simulink model "GreenCraneModel_Adjusted_110225"  (R2024b)
settings: Solver=VariableStepAuto  StartTime=0.0  StopTime=60  RelTol=1e-5
model workspace (MATLAB code in the model file):
  | %% hydralic
  | %liqud data
  | rho_l = 850;
  | 
  | %Pressure
  | Ps = 108; %bar
  | 
  | %valve data
  | pRat = 30e5; %rated pressure
  | Cd = 0.6; %discarge coefficient
  | QRat = 270/6e4;
  | Admax = QRat/Cd/(2/rho_l*pRat/2)^0.5;
  | %% multibody
  | %Cylinder 1
  | sC_1 = 0.45; %Stroke
  | L0C_1 = 0.4; %Deadlength
  | x0C_1 = 0.0; %Initial position
  | dC_1 = 0.065; %Piston diameter
  | dRC_1 = 0.035; %Rod diameter
  | %Derived values
  | dOC_1 = dC_1 + dC_1/4; %Cylinder outer diameter
  | LC_1 = sC_1 + L0C_1/3; %Cylinder length
  | tEPC_1 = L0C_1/6; %Thickness of end plate
  | dJC_1 = L0C_1/3; %Diameter of joint
  | LJC_1 = dRC_1; %Length of joint
  | LRC_1 = sC_1 + tEPC_1; %Length of rod
  | tPC_1 = L0C_1/3; %Thickness of piston
  | AC_1 = pi*dC_1^2/4; %Piston area
  | ARC_1 = pi*dRC_1^2/4; %Rod area
  | AAC_1 = AC_1 - ARC_1; %Annulus area
  | Initial_Pos = x0C_1-0.116;
  | 
  | % crane arm
  | g=9.81;
  | theta1_init=0*pi/180;
  | thetaDot1_init=0;
  | L1=3.625;
  | rho=7800;
  | L4 = 0.229;
  | Lg4x = L1-L4/2;
  | Lg4y = 0.08157;
  | 
  | abx = 0.730-0.100-0.080; %0.550; %730-100-80
  | aby = (0.223-0.075); %-0.130; %0.223-75
  | g = 9.81;
  | G1 =100*g;
  | G4 = (4*76+16)*g;
  | 
  | G = 440*g; %440*g; %447.10945
  | Gx = 3.03499; %3.03499; %3.03499
  | Gy = 0.140; %0.2; %0.06071
  | 
  | Cy = -1.040;
  | Cx = 0.427;
  | ang_CA = atan2(Cy,Cx);
  | ang_k = atan2(aby,abx);
  | b = abs(sqrt(Cy^2+Cx^2));
  | c = abs(sqrt(abx^2+aby^2)); %56.73
  | % FBD Calculations
  | %syms Ax Ay P gamma beta ang_C ang_AB r_cb r_ab L3(i) w_A w_C VBx VBy Vp crs_abp
  | L3_min = 0.772;
  | L3 = L3_min+Initial_Pos; %0.5*(x-1)/(1000-1) + 0.772;  %.172*sin(X)/1 + 0.772+0.175 0;
  | 
  | ang_C = acos((L3^2+b^2-c^2)/(2*L3*b));
  | beta = ang_CA + pi - ang_C;
  | 
  | bx = L3*cos(beta) + Cx;
  | by = L3*sin(beta) + Cy;
  | ang_AB =atan2(by,bx);
  | gamma = ang_AB + ang_k;
  | 
  | r_cb = [L3*cos(beta);L3*sin(beta);0];
  | r_ab = [bx; by; 0 ];
  | 
  | 
  | crs_abp = cross(r_ab, [cos(beta); sin(beta);0]);
  | matrix = [1, 0, cos(beta);
  |           0, 1, sin(beta);
  |           0, 0, r_ab(1)*sin(beta) - r_ab(2)*cos(beta)];
  | right = [0;(G1+G4);G*(Gx*cos(gamma)-Gy*sin(gamma))];%(G1*cos(gamma)*L1/2+G4*(cos(gamma)*Lg4x-sin(gamma)*Lg4y))
  | 
  | ANS = inv(matrix)*right;
  | Ax = ANS(1);
  | Ay = ANS(2);
  | Fl  = ANS(3); %N
  | 
  | 
  | %% FF
  | dP_0 = 7e5; %Pressure drop with comp
  | phi = 0.7130;
  | A = AC_1; % Area piston side
  | Ar = AAC_1; % Area rod side
  | BW = 0; % deadband
  | SpoolTravel = 7; % Maximum Spool Travel
  | a = (SpoolTravel-BW)/25; % Valve Slope Characteristic [mm/(L/min)]
  | 
  | %deadband
  | DeadUp = 0.13;
  | DeadDown = 0.12;
  | 
  | %% Friction force from script
  |    F_friction = 1133.4; %N
  | 
  | %% Spool travel
  | 
  | 
  | 
  | % Down
  |     U_down_vec = [0, DeadDown ,0.2, 0.4, 0.6, 0.7, 0.8, 1.0];
  |     K_down = [1e-5,1e-5,0.75,2.17,3.39,3.99,4.55,4.84]/(6e4 * sqrt(1e5));
  |     Ad_down = (K_down/(Cd*sqrt(2/rho_l))) *1e6; %mm^2
  |     Ad_down2 = 1.5*Ad_down;
  |     Ad_max_PA = 8.76; %mm^2
  |     Ad_max_BT = 1.2*Ad_max_PA;
  |     Ad_max_PB = 8.76; %mm^2
  |     Ad_max_AT = Ad_max_PB;
  | %     Dp_down_vec = [21.20, 32.96, 43.85, 48.10, 60.36]*1e5; %Pa pressure drop
  | %     VFR_down = [-3.55, -4.47, -5.18, -5.62, -6.191;
  | %            -9.95, -12.14, -14.83, -15.42, -18.60;
  | %            -14.10, -18.67, -22.17, -23.27, -27.33;
  | %            -16.96, -22.28, -27.57, -27.55, -33.1;
  | %            -17.88, -23.71, -29.04, -31.04, -35.92;
  | %            -20.53, -26.74, -32.73, -35.00, -37.53]/6e4; %m^3/s Flow
  | %     for i = 1:length(Dp_down_vec)
  | %         for j = 1:length(U_down_vec)
  | %         OAV_6x5 = sqrt( (VFR_down(i,j)).^2./(Cd^2*Dp_down_vec(i)*2/rho_l)  );
  | %         end
  | %     end
  | %
  | %
  | % % Up
  |     U_up_vec = [0, DeadUp ,0.2, 0.4, 0.6, 0.7, 0.8, 1.0];
  |     K_up = [1e-5,1e-5,0.78,2.29,3.42,4.59,5.09,5.71]/(6e4 * sqrt(1e5));
  |     Ad_up = (K_up/(Cd*sqrt(2/rho_l))) *1e6; %mm^2
  | %     Dp_up_vec = [17.39, 28.25, 36.01, 42.60, 56.50];
  | %     VFR_up = [3.36, 4.38, 4.90, 5.43, 5.86;
  | %               10.08, 12.24, 14.15, 15.51, 18.16;
  | %               9.25, 18.98, 22.92, 24.74, 27.65;
  | %               19.56, 24.95, 26.61, 29.47, 34.19;
  | %               14.84, 26.72, 32.17, 33.89, 38.51;
  | %               24.92, 26.56, 34.56, 38.50, 37.29];
  | %
  | 
  | %% motion ref
  | Amp = 0.1;
  | Mean = Amp;
values from neighbouring files (symbols this model uses):
  N = [Fl-Ffr ... (first row only)    [fyske_parametere.m]
  X = X_data.("<fPistonPosition_G_OPCfPistonPosition>")    [friksjon.m]    (also in fyske_parametere.m = M\N)
undefined symbols (not defined in the file or in its folder): Y, Z
libraries: sm_lib x35, fl_lib x31, nesl_utility x23, SimscapeFluids_lib x10, slpidlib x1
(part 1 of 3)
settings Model: Creator=Emila  LastModifiedBy=Emil
settings RTWCC: GPUComputeCapability=3.5
settings ConfigComp: PLC_OutputDir=Skrivebord  PLC_TargetIDE=twincat3  PLC_MultiTBSigbuilderTimeRange=off  PLC_FoldFBCallOutputVar=off  PLC_RemoveUnusedSSMethodCallArguments=off  PLC_UseCallOutputArgSyntax=off  PLC_EnableUnsignedAndDoubleTypes=off  PLC_EnableUDTSplitting=off  PLC_MaxFieldsInUDT=500  PLC_InlineEnumCastFunction=off

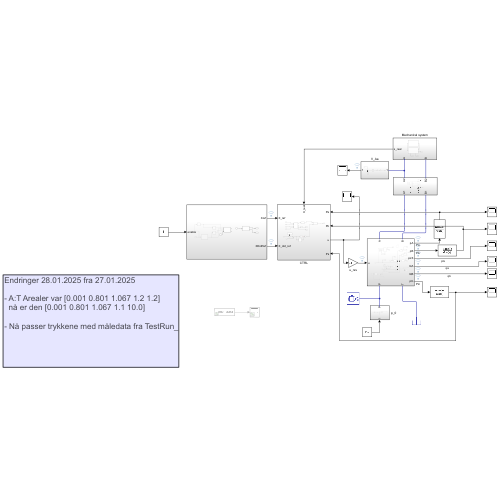
[thumbnail: Simulink's stored preview of the top-level diagram]
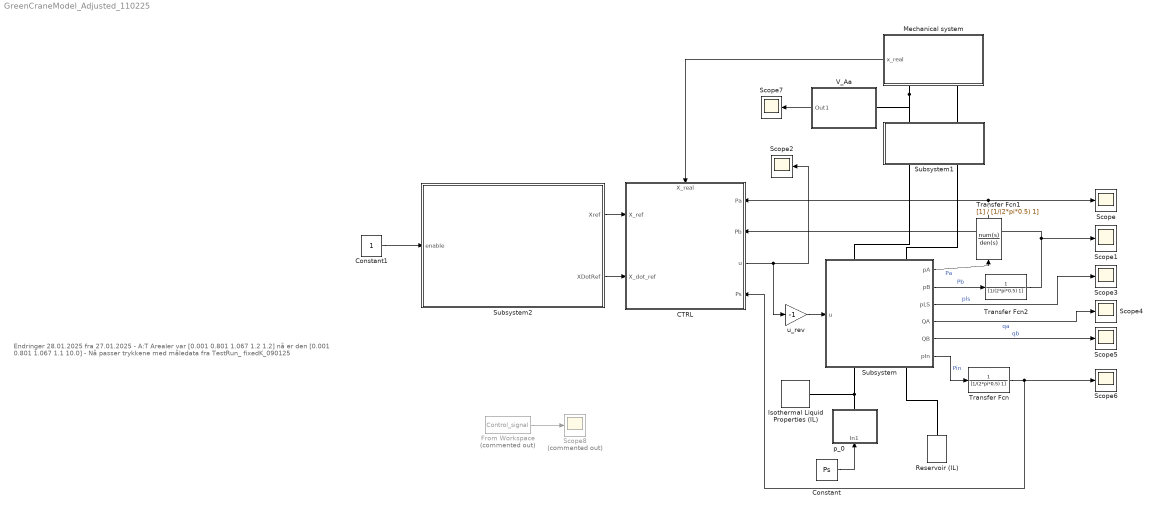
== system GreenCraneModel_Adjusted_110225 ==
  note: Endringer 28.01.2025 fra 27.01.2025
      |
      | - A:T Arealer var [0.001 0.801 1.067 1.2 1.2]
      |   nå er den [0.001 0.801 1.067 1.1 10.0]
      |
      | - Nå passer trykkene med måledata fra TestRun_ fixedK_090125
  CTRL : Subsystem
      settings: PortSchema="{\"entries\":[{\"content\":{\"sides\":[{\"content\":{\"connectorIds\":[\"In1\",\"In2\"]},\"type\":\"ConnectorPlacement.EquallySpacedRectSide\",\"uuid\":\"e7dc98bc-0c39-42fc-9d44-5c528a861935\"},{\"content\":{\"connectorIds\":[\"In4\",\"In5\",\"Out1\",\"In6\"],\"side\":\"RIGHT\"},\"type\":\"ConnectorPlacement.EquallySpacedRectSide\",\"uuid\":\"7a7fb2e4-7f4e-4840-80a8-3a9723ecfbf6\"},{\"content\":{\"connectorIds\":[\"In3\"],\"side\":\"TOP\"},\"type\":\"ConnectorPlacement.EquallySpacedRectSide\",\"uuid\":\"8314552e-40ce-493a-a910-ea6a3ee6c4fc\"}]},\"type\":\"ConnectorPlacement.EquallySpacedConnector\",\"uuid\":\"904788e7-187d-4514-a00a-56ca1dbc298c\"}],\"packageUris\":[\"http://schema.mathworks.com/mf0/Connector/R2020b\"],\"version\":\"1.0\"}"
  Constant : Constant  Value=Ps
  Constant1 : Constant
  From Workspace : FromWorkspace  Commented=on  VariableName=Control_signal  SampleTime=-1
  Isothermal Liquid Properties (IL) : fl_lib/Isothermal Liquid/Utilities/Isothermal Liquid Properties (IL)  rho_L_atm=rho_l kg/m^3  bulk_modulus_model=foundation.enum.bulk_modulus_model.const  beta_gain=6  beta_L_atm=2.1791e9 Pa  nu_atm=1.0034e-6 m^2/s  p_atm=0.101325 MPa  p_min=1 Pa  properties_range_check=simscape.enum.assert.action.error  air_fraction=0.005  polytropic_index=1.0  rho_g_atm=1.225 kg/m^3  air_dissolution_model=false  p_crit=3 MPa
  Mechanical system : Subsystem
      settings: PortSchema="{\"entries\":[{\"content\":{\"sides\":[{\"content\":{},\"type\":\"ConnectorPlacement.EquallySpacedRectSide\",\"uuid\":\"e7d79fdb-c1af-44b7-bd08-96b300e6958a\"},{\"content\":{\"connectorIds\":[\"RConn1\",\"RConn2\"],\"side\":\"RIGHT\"},\"type\":\"ConnectorPlacement.EquallySpacedRectSide\",\"uuid\":\"9182fec9-179c-4b8b-a801-95a4bf7282c9\"},{\"content\":{\"connectorIds\":[\"Out1\"],\"side\":\"TOP\"},\"type\":\"ConnectorPlacement.EquallySpacedRectSide\",\"uuid\":\"910325c5-b244-4f4d-b947-94cfd0509a86\"}]},\"type\":\"ConnectorPlacement.EquallySpacedConnector\",\"uuid\":\"3b4ea8e7-81a3-45c9-bfcb-55ef2a8eba89\"}],\"packageUris\":[\"http://schema.mathworks.com/mf0/Connector/R2020b\"],\"version\":\"1.0\"}"
  Reservoir (IL) : fl_lib/Isothermal Liquid/Elements/Reservoir (IL)  reservoir_type=foundation.enum.constant_controlled.constant  pressure_spec=foundation.enum.pressure_spec.atmospheric  reservoir_pressure=0.101325 MPa
  Scope{,1..7} (8 alike) : Scope
  Scope8 : Scope  Commented=on
  Subsystem : Subsystem
      settings: PortSchema="{\"entries\":[{\"content\":{\"sides\":[{\"content\":{\"connectorIds\":[\"In1\"]},\"type\":\"ConnectorPlacement.EquallySpacedRectSide\",\"uuid\":\"2106b7c6-6d92-4a39-9b3d-8951ce8b04e8\"},{\"content\":{\"connectorIds\":[\"Out1\",\"Out2\",\"Out3\",\"Out4\",\"Out5\",\"Out6\"],\"side\":\"RIGHT\"},\"type\":\"ConnectorPlacement.EquallySpacedRectSide\",\"uuid\":\"760f4e6f-1347-4e69-a63e-1f73879098bb\"},{\"content\":{\"connectorIds\":[\"LConn1\",\"LConn2\"],\"side\":\"TOP\"},\"type\":\"ConnectorPlacement.EquallySpacedRectSide\",\"uuid\":\"9e6a4ebb-fb50-453b-b1c2-4c0835e6495a\"},{\"content\":{\"connectorIds\":[\"RConn1\",\"RConn2\"],\"side\":\"BOTTOM\"},\"type\":\"ConnectorPlacement.EquallySpacedRectSide\",\"uuid\":\"fda93e11-89cc-40b0-95ae-4a4fae923076\"}]},\"type\":\"ConnectorPlacement.EquallySpacedConnector\",\"uuid\":\"37d72eb9-77aa-495f-a16f-a1eebb071270\"}],\"packageUris\":[\"http://schema.mathworks.com/mf0/Connector/R2020b\"],\"version\":\"1.0\"}"
  Subsystem1 : Subsystem
      settings: PortSchema="{\"entries\":[{\"content\":{\"sides\":[{\"content\":{},\"type\":\"ConnectorPlacement.EquallySpacedRectSide\",\"uuid\":\"a9f0eaf7-f148-41af-883d-8aedf66e3fe7\"},{\"content\":{\"side\":\"RIGHT\"},\"type\":\"ConnectorPlacement.EquallySpacedRectSide\",\"uuid\":\"b7d06a0e-217c-4594-9653-b1704beb7fcf\"},{\"content\":{\"connectorIds\":[\"LConn1\",\"LConn2\"],\"side\":\"TOP\"},\"type\":\"ConnectorPlacement.EquallySpacedRectSide\",\"uuid\":\"8b0b6e4d-8977-4f79-be82-c14ccdce2671\"},{\"content\":{\"connectorIds\":[\"RConn1\",\"RConn2\"],\"side\":\"BOTTOM\"},\"type\":\"ConnectorPlacement.EquallySpacedRectSide\",\"uuid\":\"d5bd5d30-b17c-4999-a2e1-ca2e0a57ee34\"}]},\"type\":\"ConnectorPlacement.EquallySpacedConnector\",\"uuid\":\"f712f636-cf3b-4e26-b860-5f0ebbe71685\"}],\"packageUris\":[\"http://schema.mathworks.com/mf0/Connector/R2020b\"],\"version\":\"1.0\"}"
  Subsystem2 : Subsystem
  Transfer Fcn : TransferFcn  Denominator=[1/(2*pi*0.5) 1]
  Transfer Fcn1 : TransferFcn  Denominator=[1/(2*pi*0.5) 1]
  Transfer Fcn2 : TransferFcn  Denominator=[1/(2*pi*0.5) 1]
  V_Aa : Subsystem
  p_0 : Subsystem
      settings: PortSchema="{\"entries\":[{\"content\":{\"sides\":[{\"content\":{\"connectorIds\":[\"LConn1\"]},\"type\":\"ConnectorPlacement.EquallySpacedRectSide\",\"uuid\":\"c4662dc8-9dce-4e03-a503-caebb8aa604d\"},{\"content\":{\"connectorIds\":[\"In1\"],\"side\":\"RIGHT\"},\"type\":\"ConnectorPlacement.EquallySpacedRectSide\",\"uuid\":\"29be6a65-4201-4b09-abee-03d6b9c83b9e\"},{\"content\":{\"side\":\"TOP\"},\"type\":\"ConnectorPlacement.EquallySpacedRectSide\",\"uuid\":\"b7c22780-7148-4981-a76e-0df66b5436d6\"},{\"content\":{\"side\":\"BOTTOM\"},\"type\":\"ConnectorPlacement.EquallySpacedRectSide\",\"uuid\":\"0d33656d-2c34-499b-a6f6-06036ba0bd38\"}]},\"type\":\"ConnectorPlacement.EquallySpacedConnector\",\"uuid\":\"6213fc7c-057e-48b9-b0cb-4c92532ae427\"}],\"packageUris\":[\"http://schema.mathworks.com/mf0/Connector/R2020b\"],\"version\":\"1.0\"}"
  u_rev : Gain  Gain=-1
  wires:
  V_Aa/1(Out1) -> Scope7/1
  Subsystem/1(pA) -> Transfer Fcn1/1  "Pa"
  Constant/1 -> p_0/1(In1)
  Subsystem/2(pB) -> Transfer Fcn2/1  "Pb"
  CTRL/1(u) -> Scope2/1, u_rev/1
  Subsystem/6(pIn) -> Transfer Fcn/1  "Pin"
  Mechanical system/1(x_real) -> CTRL/3(X_real)
  Subsystem/3(pLS) -> Scope3/1  "pls"
  Subsystem/5(QB) -> Scope5/1  "qb"
  Subsystem/4(QA) -> Scope4/1  "qa"
  Transfer Fcn/1 -> CTRL/6(Ps), Scope6/1
  Transfer Fcn2/1 -> CTRL/5(Pb), Scope1/1
  Transfer Fcn1/1 -> CTRL/4(Pa), Scope/1
  Subsystem2/1(Xref) -> CTRL/1(X_ref)
  Subsystem2/2(XDotRef) -> CTRL/2(X_dot_ref)
  Constant1/1 -> Subsystem2/1(enable)
  u_rev/1 -> Subsystem/1(u)
  From Workspace/1 -> Scope8/1
  connections:
  Mechanical system/RConn1 -- Subsystem1/LConn1 -- V_Aa/LConn1
  p_0/LConn1 -- Subsystem/RConn1 -- Isothermal Liquid Properties (IL)/RConn1
  Subsystem/LConn1 -- Subsystem1/RConn1
  Subsystem/LConn2 -- Subsystem1/RConn2
  Subsystem1/LConn2 -- Mechanical system/RConn2
  Reservoir (IL)/LConn1 -- Subsystem/RConn2

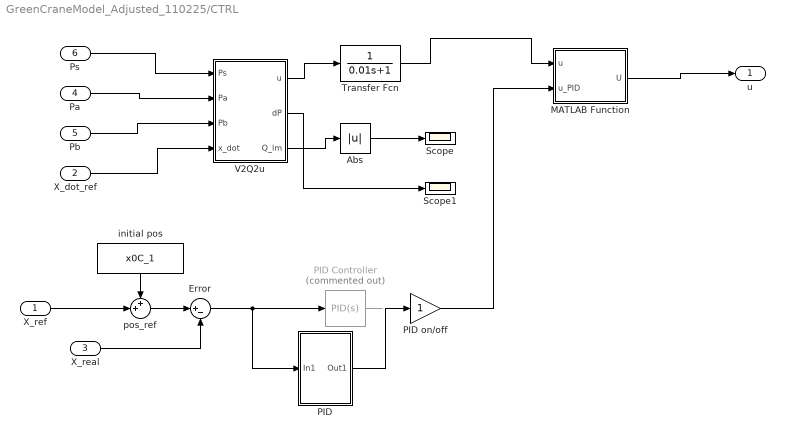
== system GreenCraneModel_Adjusted_110225/CTRL ==
  X_ref : Inport
  X_dot_ref : Inport  Port=2
  X_real : Inport  Port=3
  Pa : Inport  Port=4
  Pb : Inport  Port=5
  Ps : Inport  Port=6
  Abs : Abs  SaturateOnIntegerOverflow=off
  Error : Sum  Inputs=|+-
  MATLAB Function : MATLAB Function  TreatAsAtomicUnit=on
  PID : Subsystem
  PID Controller : slpidlib/PID Controller  Commented=on  Controller=PID  Form=Parallel  TimeDomain=Continuous-time  UseExternalTs=off  SampleTime=-1  IntegratorMethod=Forward Euler  FilterMethod=Forward Euler  ControllerParametersSource=internal  P=5  I=1  UseKiTs=off  D=1  UseExternalDerivativeSource=off  N=1e10  UseFilter=on  TunerSelectOption=Transfer Function Based (PID Tuner App)  InitialConditionSource=internal  InitialConditionForIntegrator=0  InitialConditionForFilter=0  DifferentiatorICPrevScaledInput=0  ExternalReset=none  TrackingMode=off  Kt=1  LimitOutput=off  SatLimitsSource=internal  UpperSaturationLimit=inf  LowerSaturationLimit=-inf  LinearizeAsGain=on  AntiWindupMode=none  Kb=1  LimitIntegrator=off  UpperIntegratorSaturationLimit=inf  LowerIntegratorSaturationLimit=-inf  POutMin=[]  POutMax=[]  IOutMin=[]  IOutMax=[]  DOutMin=[]  DOutMax=[]  NOutMin=[]  NOutMax=[]  SumOutMin=[]  SumOutMax=[]  SaturationOutMin=[]  SaturationOutMax=[]  PParamMin=[]  PParamMax=[]  IParamMin=[]  IParamMax=[]  DParamMin=[]  DParamMax=[]  NParamMin=[]  NParamMax=[]  KbParamMin=[]  KbParamMax=[]  KtParamMin=[]  KtParamMax=[]  KbOutMin=[]  KbOutMax=[]  KtOutMin=[]  KtOutMax=[]  IntegratorOutMin=[]  IntegratorOutMax=[]  FilterOutMin=[]  FilterOutMax=[]  SumI1OutMin=[]  SumI1OutMax=[]  SumI2OutMin=[]  SumI2OutMax=[]  SumI3OutMin=[]  SumI3OutMax=[]  SumI4OutMin=[]  SumI4OutMax=[]  SumDOutMin=[]  SumDOutMax=[]  DifferentiatorOutMin=[]  DifferentiatorOutMax=[]  FilterDiffOutCoefMin=[]  FilterDiffOutCoefMax=[]  ReciprocalOutMin=[]  ReciprocalOutMax=[]  SumDenOutMin=[]  SumDenOutMax=[]  SumNumOutMin=[]  SumNumOutMax=[]  DivideOutMin=[]  DivideOutMax=[]  UdiffTsProdOutMin=[]  UdiffTsProdOutMax=[]  NTsProdOutMin=[]  NTsProdOutMax=[]  UintegralTsProdOutMin=[]  UintegralTsProdOutMax=[]  UngainTsProdOutMin=[]  UngainTsProdOutMax=[]  ClampingZeroOutDataTypeStr=Inherit: Inherit via back propagation  ClampingZeroOutMin=[]  ClampingZeroOutMax=[]  FilterDenConstantOutDataTypeStr=Inherit: Inherit via back propagation  FilterDenConstantOutMin=[]  FilterDenConstantOutMax=[]  PCopyOutDataTypeStr=Inherit: Inherit via back propagation  PCopyOutMin=[]  PCopyOutMax=[]  NCopyOutDataTypeStr=Inherit: Inherit via back propagation  NCopyOutMin=[]  NCopyOutMax=[]  IntegratorContinuousStateAttributes=''  IntegratorStateMustResolveToSignalObject=off  IntegratorRTWStateStorageClass=Auto  FilterContinuousStateAttributes=''  FilterStateMustResolveToSignalObject=off  FilterRTWStateStorageClass=Auto  ParallelPVariant=InternalParameters  IdealPVariant=Disabled  IVariant=InternalParameters  DVariant=InternalParameters  IntegratorVariant=Continuous  SatVariant=Disabled  AWVariant=Passthrough  PCopyVariant=Disabled  TRVariant=Disabled  FdbkBlocksVariant=Forward  IdealPFdbkVariant=Disabled  SatFdbkVariant=Disabled  DerivativeFilterVariant=ContFilter  NVariant=InternalParameters  NCopyVariant=Disabled  FilterICVariant=InternalICsFilter  IntegratorICVariant=InternalICs  ExternalResetVariant=Disabled  TRSumVariant=Passthrough  SumFdbkVariant=Disabled  SumVariant=Sum_PID  TsampFilterVariant=InternalTs  TsampNgainVariant=Passthrough  TsampIntegralVariant=Disabled_SignalSpec  ExternalSaturationOutDataTypeStr=Inherit: Same as second input  DerivativeSourceVariant=ErrorSignal  PreIntVariant=InternalPreInt
  PID on/off : Gain
  Scope : Scope
  Scope1 : Scope
  Transfer Fcn : TransferFcn  Denominator=[0.01 1]
  V2Q2u : MATLAB Function  TreatAsAtomicUnit=on
  initial pos : Constant  Value=x0C_1
  pos_ref : Sum  Inputs=++|
  u : Outport
  wires:
  X_real/1 -> Error/2
  Pb/1 -> V2Q2u/3(Pb)
  Pa/1 -> V2Q2u/2(Pa)
  Ps/1 -> V2Q2u/1(Ps)
  V2Q2u/3(Q_lm) -> Abs/1
  V2Q2u/2(dP) -> Scope1/1
  X_ref/1 -> pos_ref/2
  pos_ref/1 -> Error/1
  initial pos/1 -> pos_ref/1
  V2Q2u/1(u) -> Transfer Fcn/1
  Abs/1 -> Scope/1
  PID Controller/1 -> ?
  Transfer Fcn/1 -> MATLAB Function/1(u)
  MATLAB Function/1(U) -> u/1
  PID/1(Out1) -> PID on/off/1
  Error/1 -> PID/1(In1), PID Controller/1
  X_dot_ref/1 -> V2Q2u/4(x_dot)
  PID on/off/1 -> MATLAB Function/2(u_PID)

== system GreenCraneModel_Adjusted_110225/Mechanical system ==
  Cylinder_1 : Subsystem
      settings: PortSchema="{\"entries\":[{\"content\":{\"sides\":[{\"content\":{\"connectorIds\":[\"LConn1\"]},\"type\":\"ConnectorPlacement.EquallySpacedRectSide\",\"uuid\":\"0d78c50f-9421-405f-914f-ba400f0edc4e\"},{\"content\":{\"connectorIds\":[\"RConn1\",\"Out1\"],\"side\":\"RIGHT\"},\"type\":\"ConnectorPlacement.EquallySpacedRectSide\",\"uuid\":\"3613fe88-8080-4676-8b90-d4f5ec3e9571\"},{\"content\":{\"side\":\"TOP\"},\"type\":\"ConnectorPlacement.EquallySpacedRectSide\",\"uuid\":\"fa977bd5-6674-458e-9bf8-be2185a48584\"},{\"content\":{\"connectorIds\":[\"RConn2\",\"RConn3\"],\"side\":\"BOTTOM\"},\"type\":\"ConnectorPlacement.EquallySpacedRectSide\",\"uuid\":\"b9e74392-c07a-48b0-8e27-d5ae7d883bf0\"}]},\"type\":\"ConnectorPlacement.EquallySpacedConnector\",\"uuid\":\"3e102c0d-02bf-4808-a7bf-f6d405498545\"}],\"packageUris\":[\"http://schema.mathworks.com/mf0/Connector/R2020b\"],\"version\":\"1.0\"}"
  mechanical system : Subsystem
  A : PMIOPort  Side=Right
  B : PMIOPort  Port=2  Side=Right
  x_real : Outport
  wires:
  Cylinder_1/1(x_real) -> x_real/1
  connections:
  mechanical system/LConn1 -- Cylinder_1/LConn1
  mechanical system/RConn1 -- Cylinder_1/RConn1
  B/RConn1 -- Cylinder_1/RConn3
  A/RConn1 -- Cylinder_1/RConn2

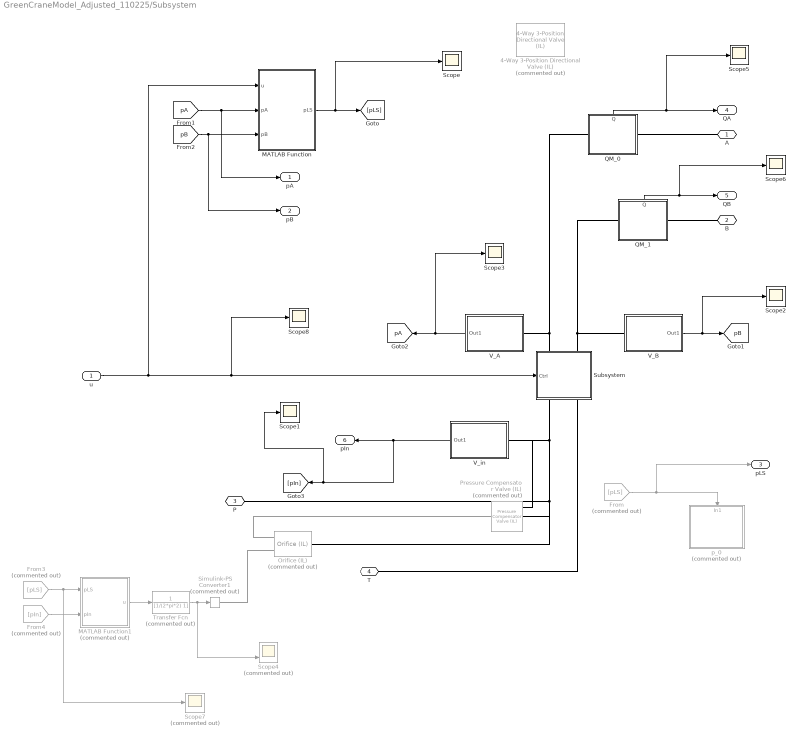
== system GreenCraneModel_Adjusted_110225/Subsystem ==
  u : Inport
  4-Way 3-Position Directional Valve (IL) : SimscapeFluids_lib/Isothermal Liquid/Valves & Orifices/Directional Control Valves/4-Way 3-Position Directional Valve (IL)  Commented=on  open_orifices_pos=fluids.isothermal_liquid.valves_orifices.directional_control_valves.enum.directional_valve_open_orifices_pos_neg.PB_AT  open_orifices_neu=fluids.isothermal_liquid.valves_orifices.directional_control_valves.enum.directional_valve_open_orifices_neutral.all_closed  open_orifices_neg=fluids.isothermal_liquid.valves_orifices.directional_control_valves.enum.directional_valve_open_orifices_pos_neg.PA_BT  neutral_assert_action=simscape.enum.assert.action.warn  area_spec=fluids.isothermal_liquid.valves_orifices.directional_control_valves.enum.directional_valve_area_spec.different  valve_spec=fluids.isothermal_liquid.valves_orifices.directional_control_valves.enum.directional_valve_spec.table1D_area_opening  del_S_max=0.005 m  area_max=1e-4 m^2  del_S_TLU=[,0, 0.114, 1] m  valve_area_TLU=[ 0.001, 0.001, 17] mm^2  del_S_vol_flow_TLU=[-0.1,0.0,0.1] m  p_diff_TLU=[-.1, .3, .5, .7] bar  vol_flow_TLU=[-1e-08, 2.2e-08, 2.8e-08, 3.4e-08; -9e-06, .00015, .0002, .00024; -.00036, .00063, .00081, .00096; -.00054, .00094, .0012, .0014; -.00091, .0016, .002, .0024] lpm  p_diff_TLU_const=[-.1, .3, .5, .7] MPa  vol_flow_TLU_const=[-.0009, .0016, .002, .0024] m^3/s  area_const=1e-4 m^2  area_leak=1e-10 m^2  area=inf m^2  Cd=Cd  Re_c=2  smoothing_factor=0.01  pressure_recovery=false  S_max_PA=-1 m  del_S_max_PA=0.005 m  area_max_PA=1e-4 m^2  del_S_TLU_PA=U_up_vec m  valve_area_TLU_PA=Ad_up mm^2  del_S_vol_flow_TLU_PA=[0, .00125, .0025, .00375, .005] m  p_diff_TLU_PA=[-.1, .3, .5, .7] MPa  vol_flow_TLU_PA=[-1e-08, 2.2e-08, 2.8e-08, 3.4e-08; -9e-06, .00015, .0002, .00024; -.00036, .00063, .00081, .00096; -.00054, .00094, .0012, .0014; -.00091, .0016, .002, .0024] m^3/s  area_const_PA=1e-4 m^2  p_diff_TLU_const_PA=[-.1, .3, .5, .7] MPa  vol_flow_TLU_const_PA=[-.0009, .0016, .002, .0024] m^3/s  S_max_PB=1 m  del_S_max_PB=0.005 m  area_max_PB=1e-4 m^2  del_S_TLU_PB=U_down_vec m  valve_area_TLU_PB=Ad_down mm^2  del_S_vol_flow_TLU_PB=[0, .00125, .0025, .00375, .005] m  p_diff_TLU_PB=[-.1, .3, .5, .7] MPa  vol_flow_TLU_PB=[-1e-08, 2.2e-08, 2.8e-08, 3.4e-08; -9e-06, .00015, .0002, .00024; -.00036, .00063, .00081, .00096; -.00054, .00094, .0012, .0014; -.00091, .0016, .002, .0024] m^3/s  area_const_PB=1e-4 m^2  p_diff_TLU_const_PB=[-.1, .3, .5, .7] MPa  vol_flow_TLU_const_PB=[-.0009, .0016, .002, .0024] m^3/s  S_max_AB=7.5e-3 m  del_S_max_AB=0.005 m  area_max_AB=1e-4 m^2  del_S_TLU_AB=[0, .00125, .0025, .00375, .005] m  valve_area_TLU_AB=[1e-10, 1e-05, 4e-05, 6e-05, .0001] m^2  del_S_vol_flow_TLU_AB=[0, .00125, .0025, .00375, .005] m  p_diff_TLU_AB=[-.1, .3, .5, .7] MPa  vol_flow_TLU_AB=[-1e-08, 2.2e-08, 2.8e-08, 3.4e-08; -9e-06, .00015, .0002, .00024; -.00036, .00063, .00081, .00096; -.00054, .00094, .0012, .0014; -.00091, .0016, .002, .0024] m^3/s  area_const_AB=1e-4 m^2  p_diff_TLU_const_AB=[-.1, .3, .5, .7] MPa  vol_flow_TLU_const_AB=[-.0009, .0016, .002, .0024] m^3/s  S_max_AT=1 m  del_S_max_AT=0.005 m  area_max_AT=1e-4 m^2  del_S_TLU_AT=U_down_vec m  valve_area_TLU_AT=Ad_down mm^2  del_S_vol_flow_TLU_AT=[0, .00125, .0025, .00375, .005] m  p_diff_TLU_AT=[-.1, .3, .5, .7] MPa  vol_flow_TLU_AT=[-1e-08, 2.2e-08, 2.8e-08, 3.4e-08; -9e-06, .00015, .0002, .00024; -.00036, .00063, .00081, .00096; -.00054, .00094, .0012, .0014; -.00091, .0016, .002, .0024] m^3/s  area_const_AT=1e-4 m^2  p_diff_TLU_const_AT=[-.1, .3, .5, .7] MPa  vol_flow_TLU_const_AT=[-.0009, .0016, .002, .0024] m^3/s  S_max_BT=-1 m  del_S_max_BT=0.005 m  area_max_BT=1e-4 m^2  del_S_TLU_BT=U_up_vec m  valve_area_TLU_BT=Ad_up mm^2  del_S_vol_flow_TLU_BT=[0, .00125, .0025, .00375, .005] m  p_diff_TLU_BT=[-.1, .3, .5, .7] MPa  vol_flow_TLU_BT=[-1e-08, 2.2e-08, 2.8e-08, 3.4e-08; -9e-06, .00015, .0002, .00024; -.00036, .00063, .00081, .00096; -.00054, .00094, .0012, .0014; -.00091, .0016, .002, .0024] m^3/s  area_const_BT=1e-4 m^2  p_diff_TLU_const_BT=[-.1, .3, .5, .7] MPa  vol_flow_TLU_const_BT=[-.0009, .0016, .002, .0024] m^3/s  S_max_PT=0 m  del_S_max_PT=0.005 m  area_max_PT=1e-4 m^2  del_S_TLU_PT=[0, .00125, .0025, .00375, .005] m  valve_area_TLU_PT=[1e-10, 1e-05, 4e-05, 6e-05, .0001] m^2  del_S_vol_flow_TLU_PT=[0, .00125, .0025, .00375, .005] m  p_diff_TLU_PT=[-.1, .3, .5, .7] MPa  vol_flow_TLU_PT=[-1e-08, 2.2e-08, 2.8e-08, 3.4e-08; -9e-06, .00015, .0002, .00024; -.00036, .00063, .00081, .00096; -.00054, .00094, .0012, .0014; -.00091, .0016, .002, .0024] m^3/s
      settings: InternalSimscapePortConfiguration="{\"Bottom\":[{\"id\":\"P\",\"label\":\"P\",\"type\":\"foundation.isothermal_liquid.isothermal_liquid\"},{\"id\":\"T\",\"label\":\"T\",\"type\":\"foundation.isothermal_liquid.isothermal_liquid\"}],\"Left\":[{\"id\":\"S\",\"label\":\"S\",\"type\":\"input\"}],\"Right\":[],\"Top\":[{\"id\":\"A\",\"label\":\"A\",\"type\":\"foundation.isothermal_liquid.isothermal_liquid\"},{\"id\":\"B\",\"label\":\"B\",\"type\":\"foundation.isothermal_liquid.isothermal_liquid\"}]}"
  From : From  Commented=on  GotoTag=pLS
  From3 : From  Commented=on  GotoTag=pLS
  From4 : From  Commented=on  GotoTag=pIn
  MATLAB Function : MATLAB Function  TreatAsAtomicUnit=on
  MATLAB Function1 : MATLAB Function  Commented=on  TreatAsAtomicUnit=on
  Orifice (IL) : SimscapeFluids_lib/Isothermal Liquid/Valves & Orifices/Orifices/Orifice (IL)  Commented=on  orifice_type=foundation.enum.constant_variable.variable  constant_orifice_spec=fluids.isothermal_liquid.valves_orifices.orifices.enum.constant_orifice_spec.area  variable_orifice_spec=fluids.isothermal_liquid.valves_orifices.orifices.enum.orifice_spec.linear  orifice_area_constant=1e-3 m^2  p_diff_TLU_constant=[-4, -3, -2, -1, -.5, 0, .5, 1, 2, 3, 4] MPa  vol_flow_TLU_constant=[-2.44, -2.12, -1.68, -1.22, -.84, 0, .85, 1.21, 1.7, 2.09, 2.41] .* 1e-3 m^3/s  S_min=0 m  del_S=1 m  open_orientation=fluids.isothermal_liquid.valves_orifices.orifices.enum.orifice_orientation.positive  area_max=200 mm^2  area_leak=1e-10 m^2  S_TLU=[0, .002, .004, .007, .017] m  orifice_area_TLU=[1e-09, 2.0352e-07, 4.0736e-05, .00011438, .00034356] m^2  area=inf m^2  Cd=0.64  Re_c=150  smoothing_factor=0.01  pressure_recovery=false  S_vol_flow_TLU=[0, .002, .004, .007, .017] m  p_diff_TLU=[.3, .5, .7] MPa  vol_flow_TLU=1e-3 * [1.7e-05, 2e-05, 2.6e-05; .0035, .0045, .0053; .7, .9, 1.06; 1.96, 2.5, 3; 6, 7.7, 9.13] m^3/s
      settings: InternalSimscapePortConfiguration="{\"Bottom\":[],\"Left\":[{\"id\":\"A\",\"label\":\"A\",\"type\":\"foundation.isothermal_liquid.isothermal_liquid\"},{\"id\":\"S\",\"label\":\"S\",\"type\":\"input\"}],\"Right\":[{\"id\":\"B\",\"label\":\"B\",\"type\":\"foundation.isothermal_liquid.isothermal_liquid\"}],\"Top\":[]}"
  Pressure Compensator Valve (IL) : SimscapeFluids_lib/Isothermal Liquid/Valves & Orifices/Pressure Control Valves/Pressure Compensator Valve (IL)  Commented=on  valve_spec=fluids.isothermal_liquid.valves_orifices.enum.closed_open.open  set_pressure_spec=foundation.enum.constant_controlled.constant  opening_spec=fluids.isothermal_liquid.valves_orifices.enum.opening_spec.linear  p_set_differential=6 bar  p_range=1 bar  area_max=200 mm^2  area_leak=1e-10 m^2  p_diff_reducing_TLU=[0.2 : 0.2 : 1.2] MPa  valve_area_reducing_TLU=[1e-05, 8e-06, 6e-06, 4e-06, 2e-06, 1e-10] m^2  p_diff_relief_TLU=[0.2 : 0.2 : 1.2] MPa  valve_area_relief_TLU=[1e-10, 2e-06, 4e-06, 6e-06, 8e-06, 1e-05] m^2  area=inf m^2  Cd=0.64  Re_c=150  smoothing_factor=0.01  pressure_recovery=false  opening_dynamics=false  tau=0.1 s
      settings: InternalSimscapePortConfiguration="{\"Bottom\":[],\"Left\":[{\"id\":\"A\",\"label\":\"A\",\"type\":\"foundation.isothermal_liquid.isothermal_liquid\"}],\"Right\":[{\"id\":\"X\",\"label\":\"X\",\"type\":\"foundation.isothermal_liquid.isothermal_liquid\"},{\"id\":\"B\",\"label\":\"B\",\"type\":\"foundation.isothermal_liquid.isothermal_liquid\"},{\"id\":\"Y\",\"label\":\"Y\",\"type\":\"foundation.isothermal_liquid.isothermal_liquid\"}],\"Top\":[]}"
  QM_0 : Subsystem
      settings: PortSchema="{\"entries\":[{\"content\":{\"sides\":[{\"content\":{\"connectorIds\":[\"LConn1\"]},\"type\":\"ConnectorPlacement.EquallySpacedRectSide\",\"uuid\":\"01703c7c-539b-4a39-97b4-ca20cf514892\"},{\"content\":{\"connectorIds\":[\"RConn1\"],\"side\":\"RIGHT\"},\"type\":\"ConnectorPlacement.EquallySpacedRectSide\",\"uuid\":\"51017cc5-2117-42de-a5e0-90b02f9996a9\"},{\"content\":{\"connectorIds\":[\"Out1\"],\"side\":\"TOP\"},\"type\":\"ConnectorPlacement.EquallySpacedRectSide\",\"uuid\":\"4a196f7b-06d4-4bc6-87ed-8d180f765f14\"}]},\"type\":\"ConnectorPlacement.EquallySpacedConnector\",\"uuid\":\"55548dd5-82ba-4402-a59b-838a9273f9a4\"}],\"packageUris\":[\"http://schema.mathworks.com/mf0/Connector/R2020b\"],\"version\":\"1.0\"}"
  QM_1 : Subsystem
      settings: PortSchema="{\"entries\":[{\"content\":{\"sides\":[{\"content\":{\"connectorIds\":[\"LConn1\"]},\"type\":\"ConnectorPlacement.EquallySpacedRectSide\",\"uuid\":\"01703c7c-539b-4a39-97b4-ca20cf514892\"},{\"content\":{\"connectorIds\":[\"RConn1\"],\"side\":\"RIGHT\"},\"type\":\"ConnectorPlacement.EquallySpacedRectSide\",\"uuid\":\"51017cc5-2117-42de-a5e0-90b02f9996a9\"},{\"content\":{\"connectorIds\":[\"Out1\"],\"side\":\"TOP\"},\"type\":\"ConnectorPlacement.EquallySpacedRectSide\",\"uuid\":\"4a196f7b-06d4-4bc6-87ed-8d180f765f14\"}]},\"type\":\"ConnectorPlacement.EquallySpacedConnector\",\"uuid\":\"55548dd5-82ba-4402-a59b-838a9273f9a4\"}],\"packageUris\":[\"http://schema.mathworks.com/mf0/Connector/R2020b\"],\"version\":\"1.0\"}"
  Scope{,1..3,5..6,8} (7 alike) : Scope
  Scope4 : Scope  Commented=on  NumInputPorts=2
  Scope7 : Scope  Commented=on
  Simulink-PS Converter1 : nesl_utility/Simulink-PS Converter  Commented=on  PhysicalDomain=network_engine_domain  SubClassName=ps_input  LeftPortType=input  RightPortType=output  PseudoPeriodic=off  Frequencies=[]  NoiseDistribution=none  NoiseParameters=[]  Unit=1  AffineConversion=off  FilteringAndDerivatives=filter  SimscapeFilterOrder=2  InputFilterTimeConstant=0.001  UdotUserProvided=0
  Subsystem : Subsystem
      settings: PortSchema="{\"entries\":[{\"content\":{\"sides\":[{\"content\":{\"connectorIds\":[\"In1\"]},\"type\":\"ConnectorPlacement.EquallySpacedRectSide\",\"uuid\":\"6993dbde-6cba-46a2-b1d5-f1047b136426\"},{\"content\":{\"side\":\"RIGHT\"},\"type\":\"ConnectorPlacement.EquallySpacedRectSide\",\"uuid\":\"3ad9b2a3-36be-44b7-a33f-fa48c865a093\"},{\"content\":{\"connectorIds\":[\"LConn1\",\"LConn2\"],\"side\":\"TOP\"},\"type\":\"ConnectorPlacement.EquallySpacedRectSide\",\"uuid\":\"66e9811c-0a42-4ab5-bd83-e8b75281c572\"},{\"content\":{\"connectorIds\":[\"RConn1\",\"RConn2\"],\"side\":\"BOTTOM\"},\"type\":\"ConnectorPlacement.EquallySpacedRectSide\",\"uuid\":\"046bb913-9a9e-4ef9-939b-8e65f57c81b5\"}]},\"type\":\"ConnectorPlacement.EquallySpacedConnector\",\"uuid\":\"5e1ffb91-7437-41ca-a8e1-7c47f283d11a\"}],\"packageUris\":[\"http://schema.mathworks.com/mf0/Connector/R2020b\"],\"version\":\"1.0\"}"
  Transfer Fcn : TransferFcn  Commented=on  Denominator=[1/(2*pi*2) 1]
  V_A : Subsystem
  V_B : Subsystem
  V_in : Subsystem
  p_0 : Subsystem  Commented=on
      settings: PortSchema="{\"entries\":[{\"content\":{\"sides\":[{\"content\":{\"connectorIds\":[\"LConn1\"]},\"type\":\"ConnectorPlacement.EquallySpacedRectSide\",\"uuid\":\"c4662dc8-9dce-4e03-a503-caebb8aa604d\"},{\"content\":{\"side\":\"RIGHT\"},\"type\":\"ConnectorPlacement.EquallySpacedRectSide\",\"uuid\":\"29be6a65-4201-4b09-abee-03d6b9c83b9e\"},{\"content\":{\"connectorIds\":[\"In1\"],\"side\":\"TOP\"},\"type\":\"ConnectorPlacement.EquallySpacedRectSide\",\"uuid\":\"b7c22780-7148-4981-a76e-0df66b5436d6\"}]},\"type\":\"ConnectorPlacement.EquallySpacedConnector\",\"uuid\":\"6213fc7c-057e-48b9-b0cb-4c92532ae427\"}],\"packageUris\":[\"http://schema.mathworks.com/mf0/Connector/R2020b\"],\"version\":\"1.0\"}"
  A : PMIOPort  Side=Left
  B : PMIOPort  Port=2  Side=Left
  P : PMIOPort  Port=3  Side=Right
  T : PMIOPort  Port=4  Side=Right
  pA : Outport
  pB : Outport  Port=2
  pLS : Outport  Port=3
  QA : Outport  Port=4
  QB : Outport  Port=5
  pIn : Outport  Port=6
  tag scope: pA=global, pB=global
  wires:
  u/1 -> MATLAB Function/1(u), Subsystem/1(Ctrl), Scope8/1
  QM_0/1(Q) -> Scope5/1, QA/1
  From/1 -> pLS/1, p_0/1(In1)
  V_A/1(Out1) -> Scope3/1, [pA]
  V_B/1(Out1) -> Scope2/1, [pB]
  [pA] -> pA/1, MATLAB Function/2(pA)
  [pB] -> pB/1, MATLAB Function/3(pB)
  MATLAB Function/1(pLS) -> Scope/1, [pLS]
  QM_1/1(Q) -> Scope6/1, QB/1
  V_in/1(Out1) -> Scope1/1, [pIn], pIn/1
  From4/1 -> MATLAB Function1/2(pIn)
  From3/1 -> Scope7/1, MATLAB Function1/1(pLS)
  Transfer Fcn/1 -> Scope4/2, Simulink-PS Converter1/1
  MATLAB Function1/1(u) -> Transfer Fcn/1
  connections:
  A/RConn1 -- QM_0/RConn1
  P/RConn1 -- Orifice (IL)/RConn1 -- Pressure Compensator Valve (IL)/RConn2 -- Subsystem/RConn1 -- Pressure Compensator Valve (IL)/RConn1 -- V_in/LConn1
  B/RConn1 -- QM_1/RConn1
  V_B/LConn1 -- Subsystem/LConn2 -- QM_1/LConn1
  V_A/LConn1 -- QM_0/LConn1 -- Subsystem/LConn1
  Orifice (IL)/LConn1 -- Pressure Compensator Valve (IL)/LConn1
  Subsystem/RConn2 -- T/RConn1
  Simulink-PS Converter1/RConn1 -- Orifice (IL)/LConn2

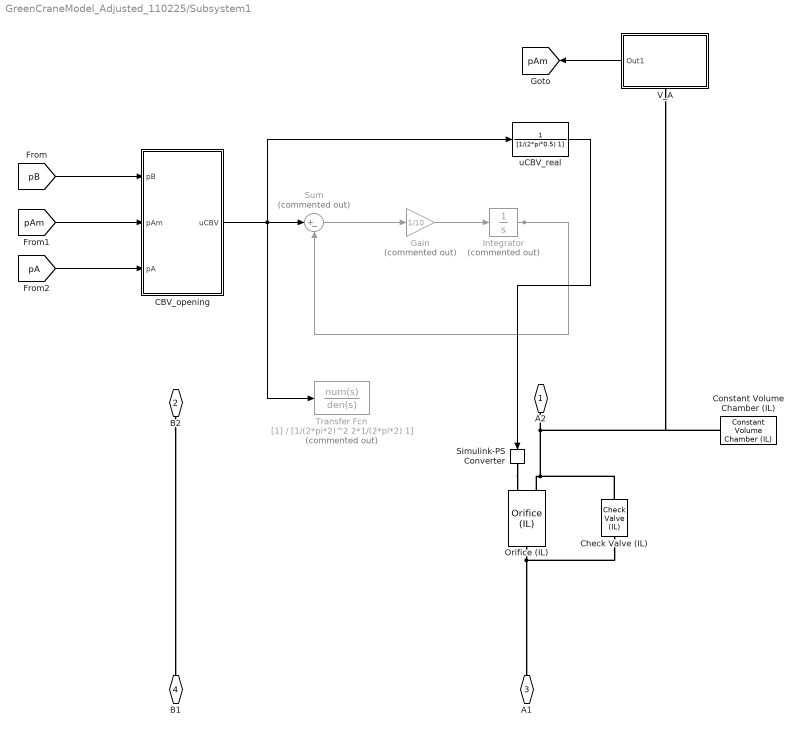
== system GreenCraneModel_Adjusted_110225/Subsystem1 ==
  CBV_opening : MATLAB Function  TreatAsAtomicUnit=on
  Check Valve (IL) : SimscapeFluids_lib/Isothermal Liquid/Valves & Orifices/Directional Control Valves/Check Valve (IL)  opening_spec=fluids.isothermal_liquid.valves_orifices.enum.PressureOpeningSpec.Linear  pressure_control_spec=fluids.isothermal_liquid.valves_orifices.enum.pressure_control_spec.dp  p_crack_differential=0.2 bar  p_crack_gauge=0.1 MPa  press_max_differential=3 bar  press_max_gauge=0.2 MPa  area_max=6 mm^2  area_leak=1e-10 m^2  p_diff_TLU=[0.01 : 0.01 : 0.1] MPa  valve_area_TLU=[1e-10, 1e-05, 2e-05, 3e-05, 4e-05, 5e-05, 6e-05, 7.5e-05, 8.5e-05, .0001] m^2  vol_flow_TLU=[.000358, .045, .11, .191, .284, .39, .505, .63, .764, .905] .* 1e-3 m^3/s  area=inf m^2  Cd=0.64  Re_c=150  smoothing_factor=0.01  pressure_recovery=false  opening_dynamics=false  tau=0.1 s
      settings: InternalSimscapePortConfiguration="{\"Bottom\":[],\"Left\":[{\"id\":\"A\",\"label\":\"A\",\"type\":\"foundation.isothermal_liquid.isothermal_liquid\"}],\"Right\":[{\"id\":\"B\",\"label\":\"B\",\"type\":\"foundation.isothermal_liquid.isothermal_liquid\"}],\"Top\":[]}"
  Constant Volume Chamber (IL) : fl_lib/Isothermal Liquid/Elements/Constant Volume Chamber (IL)  volume=5 l  p_I_specify=on  p_I_priority=High  p_I=70 bar  p_I_nominal_specify=off  p_I_nominal_value=1  p_I_nominal_unit=MPa
      settings: InternalSimscapePortConfiguration="{\"Bottom\":[],\"Left\":[{\"id\":\"A\",\"label\":\"A\",\"type\":\"foundation.isothermal_liquid.isothermal_liquid\"}],\"Right\":[],\"Top\":[]}"
  Gain : Gain  Commented=on  Gain=1/10
  Integrator : Integrator  Commented=on
  Orifice (IL) : SimscapeFluids_lib/Isothermal Liquid/Valves & Orifices/Orifices/Orifice (IL)  orifice_type=foundation.enum.constant_variable.variable  constant_orifice_spec=fluids.isothermal_liquid.valves_orifices.orifices.enum.constant_orifice_spec.area  variable_orifice_spec=fluids.isothermal_liquid.valves_orifices.orifices.enum.orifice_spec.linear  orifice_area_constant=1e-3 m^2  p_diff_TLU_constant=[-4, -3, -2, -1, -.5, 0, .5, 1, 2, 3, 4] MPa  vol_flow_TLU_constant=[-2.44, -2.12, -1.68, -1.22, -.84, 0, .85, 1.21, 1.7, 2.09, 2.41] .* 1e-3 m^3/s  S_min=0 m  del_S=1 m  open_orientation=fluids.isothermal_liquid.valves_orifices.orifices.enum.orifice_orientation.positive  area_max=80 mm^2  area_leak=1e-10 m^2  S_TLU=[0, .002, .004, .007, .017] m  orifice_area_TLU=[1e-09, 2.0352e-07, 4.0736e-05, .00011438, .00034356] m^2  area=inf m^2  Cd=0.64  Re_c=2  smoothing_factor=0.01  pressure_recovery=false  S_vol_flow_TLU=[0, .002, .004, .007, .017] m  p_diff_TLU=[.3, .5, .7] MPa  vol_flow_TLU=1e-3 * [1.7e-05, 2e-05, 2.6e-05; .0035, .0045, .0053; .7, .9, 1.06; 1.96, 2.5, 3; 6, 7.7, 9.13] m^3/s
      settings: InternalSimscapePortConfiguration="{\"Bottom\":[],\"Left\":[{\"id\":\"A\",\"label\":\"A\",\"type\":\"foundation.isothermal_liquid.isothermal_liquid\"},{\"id\":\"S\",\"label\":\"S\",\"type\":\"input\"}],\"Right\":[{\"id\":\"B\",\"label\":\"B\",\"type\":\"foundation.isothermal_liquid.isothermal_liquid\"}],\"Top\":[]}"
  Simulink-PS Converter : nesl_utility/Simulink-PS Converter  PhysicalDomain=network_engine_domain  SubClassName=ps_input  LeftPortType=input  RightPortType=output  PseudoPeriodic=off  Frequencies=[]  NoiseDistribution=none  NoiseParameters=[]  Unit=1  AffineConversion=off  FilteringAndDerivatives=provide  SimscapeFilterOrder=1  InputFilterTimeConstant=0.001  UdotUserProvided=0
  Sum : Sum  Commented=on  Inputs=|+-
  Transfer Fcn : TransferFcn  Commented=on  Denominator=[1/(2*pi*2)^2 2*1/(2*pi*2) 1]
  V_A : Subsystem
      settings: PortSchema="{\"entries\":[{\"content\":{\"sides\":[{\"content\":{},\"type\":\"ConnectorPlacement.EquallySpacedRectSide\",\"uuid\":\"4d44c916-36b4-4891-95d7-b71f690fb118\"},{\"content\":{\"connectorIds\":[\"Out1\"],\"side\":\"RIGHT\"},\"type\":\"ConnectorPlacement.EquallySpacedRectSide\",\"uuid\":\"b0ccc4ef-865c-4258-9950-e2b42fb6e66f\"},{\"content\":{\"side\":\"TOP\"},\"type\":\"ConnectorPlacement.EquallySpacedRectSide\",\"uuid\":\"000783d9-e516-4133-ab05-d5308326cee4\"},{\"content\":{\"connectorIds\":[\"RConn1\"],\"side\":\"BOTTOM\"},\"type\":\"ConnectorPlacement.EquallySpacedRectSide\",\"uuid\":\"39508f26-00e3-44ba-9bd3-5b0574c641a0\"}]},\"type\":\"ConnectorPlacement.EquallySpacedConnector\",\"uuid\":\"7f98e183-dea6-48a9-9217-d90bb6709085\"}],\"packageUris\":[\"http://schema.mathworks.com/mf0/Connector/R2020b\"],\"version\":\"1.0\"}"
  uCBV_real : TransferFcn  Denominator=[1/(2*pi*0.5) 1]
  A2 : PMIOPort  Side=Left
  B2 : PMIOPort  Port=2  Side=Left
  A1 : PMIOPort  Port=3  Side=Right
  B1 : PMIOPort  Port=4  Side=Right
  tag scope: pAm=global
  wires:
  V_A/1(Out1) -> [pAm]
  [pB] -> CBV_opening/1(pB)
  [pAm] -> CBV_opening/2(pAm)
  [pA] -> CBV_opening/3(pA)
  Gain/1 -> Integrator/1
  Integrator/1 -> Sum/2
  CBV_opening/1(uCBV) -> uCBV_real/1, Transfer Fcn/1, Sum/1
  Sum/1 -> Gain/1
  uCBV_real/1 -> Simulink-PS Converter/1
  connections:
  Check Valve (IL)/RConn1 -- Orifice (IL)/LConn1 -- V_A/RConn1 -- Constant Volume Chamber (IL)/LConn1 -- A2/RConn1
  Check Valve (IL)/LConn1 -- A1/RConn1 -- Orifice (IL)/RConn1
  B2/RConn1 -- B1/RConn1
  Simulink-PS Converter/RConn1 -- Orifice (IL)/LConn2

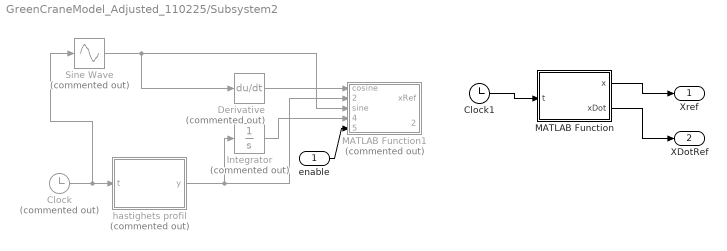
== system GreenCraneModel_Adjusted_110225/Subsystem2 ==
  enable : Inport
  Clock : Clock  Commented=on
  Clock1 : Clock
  Derivative : Derivative  Commented=on
  Integrator : Integrator  Commented=on
  MATLAB Function : MATLAB Function  TreatAsAtomicUnit=on
  MATLAB Function1 : MATLAB Function  Commented=on  TreatAsAtomicUnit=on
  Sine Wave : Sin  Commented=on  TimeSource=Use external signal  Amplitude=Amp  Bias=Mean  Frequency=0.05*2*pi  Phase=3*pi/2  SampleTime=0
  hastighets profil : MATLAB Function  Commented=on  TreatAsAtomicUnit=on
  Xref : Outport
  XDotRef : Outport  Port=2
  wires:
  Sine Wave/1 -> Derivative/1, MATLAB Function1/3(sine)
  Derivative/1 -> MATLAB Function1/1(cosine)
  hastighets profil/1(y) -> MATLAB Function1/2(ramp_vel), Integrator/1
  Clock/1 -> Sine Wave/1, hastighets profil/1(t)
  enable/1 -> MATLAB Function1/5(enable)
  Integrator/1 -> MATLAB Function1/4(ramp_pos)
  Clock1/1 -> MATLAB Function/1(t)
  MATLAB Function/1(x) -> Xref/1
  MATLAB Function/2(xDot) -> XDotRef/1

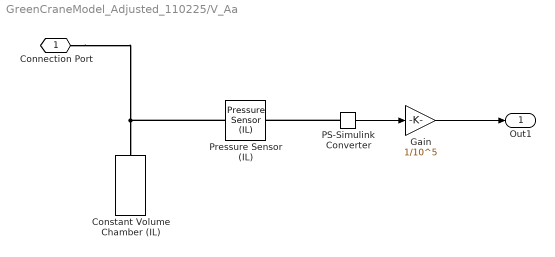
== system GreenCraneModel_Adjusted_110225/V_Aa ==
  Constant Volume Chamber (IL) : fl_lib/Isothermal Liquid/Elements/Constant Volume Chamber (IL)  volume=1 l  p_I_specify=on  p_I_priority=High  p_I=70 bar  p_I_nominal_specify=off  p_I_nominal_value=1  p_I_nominal_unit=MPa
      settings: InternalSimscapePortConfiguration="{\"Bottom\":[],\"Left\":[{\"id\":\"A\",\"label\":\"A\",\"type\":\"foundation.isothermal_liquid.isothermal_liquid\"}],\"Right\":[],\"Top\":[]}"
  Gain : Gain  Gain=1/10^5
  PS-Simulink Converter : nesl_utility/PS-Simulink Converter  PhysicalDomain=network_engine_domain  SubClassName=ps_output  LeftPortType=input  RightPortType=output  PseudoPeriodic=off  Frequencies=[]  VectorFormat=inherit  Unit=inherit  AffineConversion=off
  Pressure Sensor (IL) : fl_lib/Isothermal Liquid/Sensors/Pressure Sensor (IL)  pressure_measure=foundation.enum.pressure_measure.gauge
      settings: InternalSimscapePortConfiguration="{\"Bottom\":[],\"Left\":[{\"id\":\"A\",\"label\":\"A\",\"type\":\"foundation.isothermal_liquid.isothermal_liquid\"}],\"Right\":[{\"id\":\"Pg\",\"label\":\"Pg\",\"type\":\"output\"}],\"Top\":[]}"
  Connection Port : PMIOPort  Side=Left
  Out1 : Outport
  wires:
  Gain/1 -> Out1/1
  PS-Simulink Converter/1 -> Gain/1
  connections:
  Pressure Sensor (IL)/LConn1 -- Constant Volume Chamber (IL)/LConn1 -- Connection Port/RConn1
  PS-Simulink Converter/LConn1 -- Pressure Sensor (IL)/RConn1

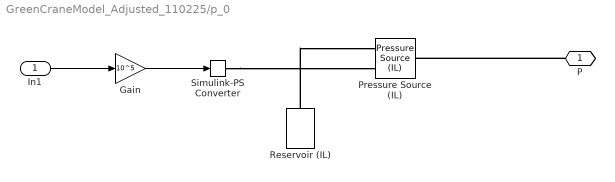
== system GreenCraneModel_Adjusted_110225/p_0 ==
  In1 : Inport
  Gain : Gain  Gain=10^5
  Pressure Source (IL) : fl_lib/Isothermal Liquid/Sources/Pressure Source (IL)  source_type=foundation.enum.constant_controlled.controlled  pressure_differential=0 MPa
      settings: InternalSimscapePortConfiguration="{\"Bottom\":[],\"Left\":[{\"id\":\"A\",\"label\":\"A\",\"type\":\"foundation.isothermal_liquid.isothermal_liquid\"},{\"id\":\"P\",\"label\":\"P\",\"type\":\"input\"}],\"Right\":[{\"id\":\"B\",\"label\":\"B\",\"type\":\"foundation.isothermal_liquid.isothermal_liquid\"}],\"Top\":[]}"
  Reservoir (IL) : fl_lib/Isothermal Liquid/Elements/Reservoir (IL)  reservoir_type=foundation.enum.constant_controlled.constant  pressure_spec=foundation.enum.pressure_spec.atmospheric  reservoir_pressure=0.101325 MPa
  Simulink-PS Converter : nesl_utility/Simulink-PS Converter  PhysicalDomain=network_engine_domain  SubClassName=ps_input  LeftPortType=input  RightPortType=output  PseudoPeriodic=off  Frequencies=[]  NoiseDistribution=none  NoiseParameters=[]  Unit=1  AffineConversion=off  FilteringAndDerivatives=provide  SimscapeFilterOrder=1  InputFilterTimeConstant=0.001  UdotUserProvided=0
  P : PMIOPort  Side=Left
  wires:
  In1/1 -> Gain/1
  Gain/1 -> Simulink-PS Converter/1
  connections:
  Reservoir (IL)/LConn1 -- Pressure Source (IL)/LConn1
  Simulink-PS Converter/RConn1 -- Pressure Source (IL)/LConn2
  P/RConn1 -- Pressure Source (IL)/RConn1

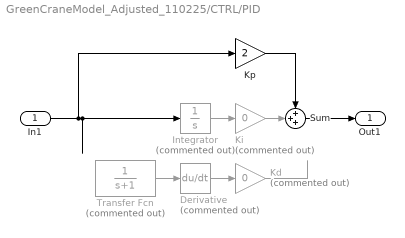
== system GreenCraneModel_Adjusted_110225/CTRL/PID ==
  In1 : Inport
  Derivative : Derivative  Commented=on
  Integrator : Integrator  Commented=on
  Kd : Gain  Commented=on  Gain=0
  Ki : Gain  Commented=on  Gain=0
  Kp : Gain  Gain=2
  Sum : Sum  Inputs=+++
  Transfer Fcn : TransferFcn  Commented=on  Denominator=[1 1]
  Out1 : Outport
  wires:
  Integrator/1 -> Ki/1
  Derivative/1 -> Kd/1
  In1/1 -> Integrator/1, Kp/1
  Sum/1 -> Out1/1
  Kd/1 -> ?
  Kp/1 -> Sum/1
  Ki/1 -> Sum/2
  Transfer Fcn/1 -> Derivative/1
